simulink model "maglev_3d"  (R2022b)
settings: Solver=VariableStepAuto  StartTime=0.0  StopTime=1  RelTol=1e-3
settings Model: Creator=hansae  LastModifiedBy=hansae

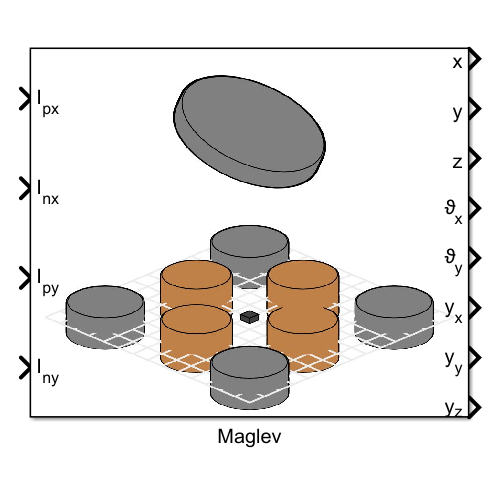
[thumbnail: Simulink's stored preview of the top-level diagram]
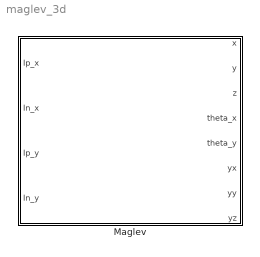
== system maglev_3d ==
  Maglev : Subsystem
      mask Display:
      | image('$imagefile'); % Use "Edit Image" on toolstrip to change.
      | 
      | port_label('input', 1, 'I_{px} ','interpreter','tex')
      | port_label('input', 2, 'I_{nx}','interpreter','tex')
      | 
      | port_label('input', 3, 'I_{py}','interpreter','tex')
      | port_label('input', 4, 'I_{ny}','interpreter','tex')
      | 
      | port_label('output', 1, 'x','interpreter','tex')
      | port_label('output', 2, 'y','interpreter','tex')
      | port_label('output', 3, 'z','interpreter','tex')
      | port_label('output', 4, '\vartheta_x','interpreter','tex')
      | port_label('output', 5, '\vartheta_y','interpreter','tex')
      | 
      | port_label('output', 6, 'y_x','interpreter','tex')
      | port_label('output', 7, 'y_y','interpreter','tex')
      | port_label('output', 8, 'y_z','interpreter','tex')

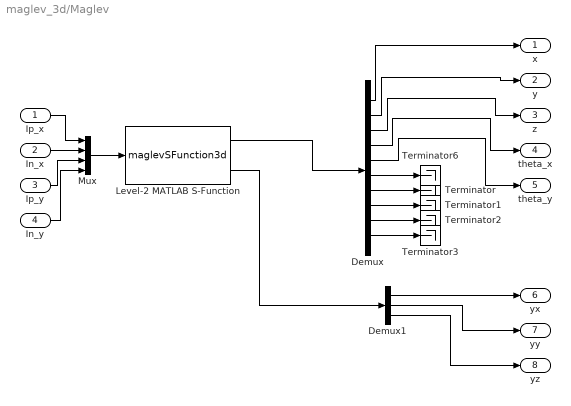
== system maglev_3d/Maglev ==
  Ip_x : Inport
  In_x : Inport  Port=2
  Ip_y : Inport  Port=3
  In_y : Inport  Port=4
  Demux : Demux  Outputs=10
  Demux1 : Demux  Outputs=3
  Level-2 MATLAB S-Function : M-S-Function  FunctionName=maglevSFunction3d
  Mux : Mux
  Terminator{,1..3,6} (5 alike) : Terminator
  x : Outport
  y : Outport  Port=2
  z : Outport  Port=3
  theta_x : Outport  Port=4
  theta_y : Outport  Port=5
  yx : Outport  Port=6
  yy : Outport  Port=7
  yz : Outport  Port=8
  wires:
  Demux/1 -> x/1
  Demux/3 -> z/1
  Demux1/1 -> yx/1
  Mux/1 -> Level-2 MATLAB S-Function/1
  Ip_x/1 -> Mux/1
  In_x/1 -> Mux/2
  Level-2 MATLAB S-Function/2 -> Demux1/1
  Level-2 MATLAB S-Function/1 -> Demux/1
  Demux/2 -> y/1
  Ip_y/1 -> Mux/3
  In_y/1 -> Mux/4
  Demux1/3 -> yz/1
  Demux1/2 -> yy/1
  Demux/10 -> Terminator3/1
  Demux/7 -> Terminator/1
  Demux/8 -> Terminator1/1
  Demux/9 -> Terminator2/1
  Demux/4 -> theta_x/1
  Demux/5 -> theta_y/1
  Demux/6 -> Terminator6/1
